simulink model "Main_ComplexTherma_Test_IGBT_Revised"  (R2022b)
settings: Solver=ode45  StartTime=0.0  StopTime=time  RelTol=1e-3  EnableMultiTasking=on
values from neighbouring files (symbols this model uses):
  C1diode = tau1diode/R1diode    (= 0.047619047619)    [fcnLE.m]
  C1igbt = tau1igbt/R1igbt    (= 0.0806451612903)    [fcnLE.m]
  C2diode = tau2diode/R2diode    (= 0.434782608696)    [fcnLE.m]
  C2igbt = tau2igbt/R2igbt    (= 0.909090909091)    [fcnLE.m]
  C3diode = tau3diode/R3diode    (= 1.27098321343)    [fcnLE.m]
  C3igbt = tau3igbt/R3igbt    (= 2.43697478992)    [fcnLE.m]
  C4diode = tau4diode/R4diode    (= 11.7824773414)    [fcnLE.m]
  C4igbt = tau4igbt/R4igbt    (= 11.8421052632)    [fcnLE.m]
  C5diode = tau5diode/R5diode    (= 237.037037037)    [fcnLE.m]
  C5igbt = tau5igbt/R5igbt    (= 219)    [fcnLE.m]
  fswitch = 10000    [fcnLE.m]
  R1diode = 0.0126    [fcnLE.m]
  R1igbt = 0.0062    [fcnLE.m]
  R2diode = 0.0391    [fcnLE.m]
  R2igbt = 0.022    [fcnLE.m]
  R3diode = 0.0417    [fcnLE.m]
  R3igbt = 0.0238    [fcnLE.m]
  R4diode = 0.0331    [fcnLE.m]
  R4igbt = 0.038    [fcnLE.m]
  R5diode = 0.0135    [fcnLE.m]
  R5igbt = 0.01    [fcnLE.m]
  R6igbt = 0.1    [fcnLE.m]
  udc = config_battery.U_sys_nom    [fcnLE.m]
undefined symbols (not defined in the file or in its folder): eqivalentCircuitParameters, eta_t, i_g, Rw, vehicle_weight
libraries: spsParallelRLCBranchLib x11, spsControlledCurrentSourceLib x2, spsVoltageMeasurementLib x2, spsDCVoltageSourceLib x1, spspowerguiLib x1
settings Model: Creator=fengqi.chang  LastModifiedBy=wangyifei
settings SolverCC: AlgebraicLoopSolver=TrustRegion
settings DataIOCC: LimitDataPoints=on  SaveFormat=Array  ReturnWorkspaceOutputs=off
settings OptimizationCC: LifeSpan=inf
settings DebuggingCC: SolverPrmCheckMsg=warning  UnconnectedInputMsg=warning  UnconnectedOutputMsg=warning  UnconnectedLineMsg=warning  SFUnexpectedBacktrackingDiag=warning  SFNoUnconditionalDefaultTransitionDiag=warning  SFExecutionAtInitializationDiag=none  SFMachineParentedDataDiag=warning  ArithmeticOperatorsInVariantConditions=warning
settings HardwareCC: ProdBitPerPointer=32  ProdBitPerSizeT=32  ProdBitPerPtrDiffT=32  ProdLargestAtomicFloat=None  ProdIntDivRoundTo=Undefined  ProdEndianess=Unspecified  ProdWordSize=32  ProdHWDeviceType=32-bit Generic
settings ModelReferenceCC: EnableRefExpFcnMdlSchedulingChecks=on  PropagateSignalLabelsOutOfModel=off
settings SFSimCC: SimUseLocalCustomCode=off  CustomCodeUndefinedFunction=UseInterfaceOnly
settings RTWCC: RTWUseLocalCustomCode=off
settings CodeAppCC: StateflowObjectComments=on
settings GRTTargetCC: TargetLangStandard=C89/C90 (ANSI)
settings ConfigComp: CovMetricSettings=dw  CovSaveCumulativeToWorkspaceVar=on  CovSaveSingleToWorkspaceVar=on  CovExternalEMLEnable=off  CovSFcnEnable=off
settings SimscapeCC: SimscapeNormalizeSystem=off

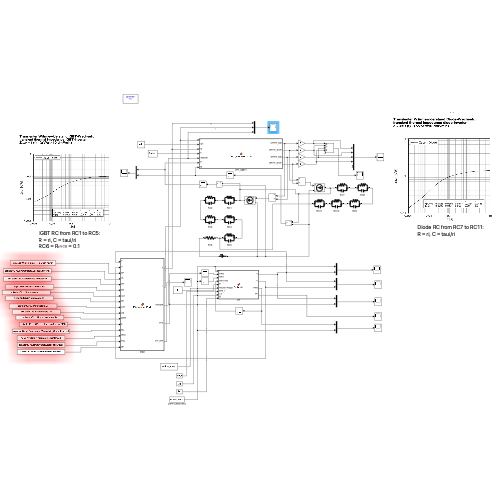
[thumbnail: Simulink's stored preview of the top-level diagram]
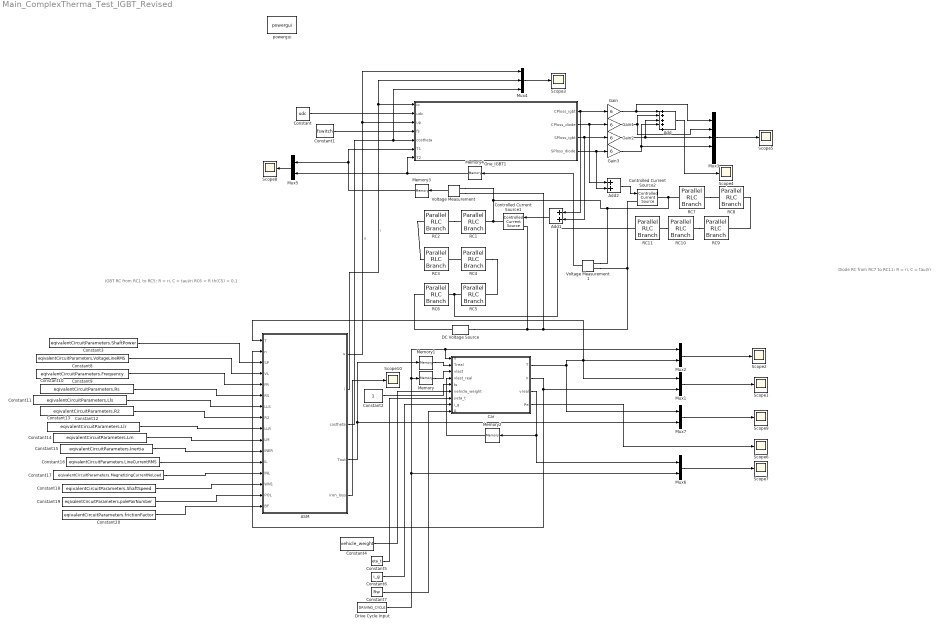
== system Main_ComplexTherma_Test_IGBT_Revised ==
  note: IGBT RC from RC1 to RC5:
      | R = ri, C = taui/ri
      | RC6 = R th(CS) = 0.1
  note: Diode RC from RC7 to RC11:
      | R = ri, C = taui/ri
  ASM : MATLAB Function  TreatAsAtomicUnit=on
  Add : Sum  Inputs=+++++
  Add1 : Sum
  Add2 : Sum
  Car : MATLAB Function  TreatAsAtomicUnit=on
  Constant : Constant  Value=udc
  Constant1 : Constant  Value=fswitch
  Constant10 : Constant  Value=eqivalentCircuitParameters.Rs
  Constant11 : Constant  Value=eqivalentCircuitParameters.Lls
  Constant12 : Constant  Value=eqivalentCircuitParameters.R2
  Constant13 : Constant  Value=eqivalentCircuitParameters.Llr
  Constant14 : Constant  Value=eqivalentCircuitParameters.Lm
  Constant15 : Constant  Value=eqivalentCircuitParameters.Inertia
  Constant16 : Constant  Value=eqivalentCircuitParameters.LineCurrentRMS
  Constant17 : Constant  Value=eqivalentCircuitParameters.MagnetizingCurrentNoLoad
  Constant18 : Constant  Value=eqivalentCircuitParameters.ShaftSpeed
  Constant19 : Constant  Value=eqivalentCircuitParameters.polePairNumber
  Constant2 : Constant
  Constant20 : Constant  Value=eqivalentCircuitParameters.frictionFactor
  Constant3 : Constant  Value=eqivalentCircuitParameters.ShaftPower
  Constant4 : Constant  Value=vehicle_weight
  Constant5 : Constant  Value=eta_t
  Constant6 : Constant  Value=i_g
  Constant7 : Constant  Value=Rw
  Constant8 : Constant  Value=eqivalentCircuitParameters.VoltageLineRMS
  Constant9 : Constant  Value=eqivalentCircuitParameters.Frequency
  Controlled Current Source1 : spsControlledCurrentSourceLib/Controlled Current Source  Initialize=on  Source_Type=AC  Amplitude=0  Phase=0  Frequency=0  Measurements=None
  Controlled Current Source2 : spsControlledCurrentSourceLib/Controlled Current Source  Initialize=on  Source_Type=AC  Amplitude=0  Phase=0  Frequency=0  Measurements=None
  DC Voltage Source : spsDCVoltageSourceLib/DC Voltage Source  Amplitude=50  Measurements=None
  Drive Cycle Input : FromWorkspace  VariableName=DRIVING_CYCLE  SampleTime=-1  OutputAfterFinalValue=Setting to zero
  Gain{,1..3} (4 alike) : Gain  Gain=6
  Memory : Memory  InheritSampleTime=on
  Memory1 : Memory  InheritSampleTime=on
  Memory2 : Memory  InheritSampleTime=on
  Memory3 : Memory  InitialCondition=25  InheritSampleTime=on
  Memory4 : Memory  InitialCondition=25  InheritSampleTime=on
  Mux{1..2,5..7} (5 alike) : Mux  Inputs=2
  Mux3 : Mux  Inputs=5
  Mux4 : Mux  Inputs=3
  One_IGBT1 : MATLAB Function  TreatAsAtomicUnit=on
  RC1 : spsParallelRLCBranchLib/Parallel RLC Branch  LConnTagsString=a  RConnTagsString=__new0  BranchType=RC  Resistance=R1igbt  Inductance=1e-3  SetiL0=off  InitialCurrent=0  Capacitance=C1igbt  Setx0=off  InitialVoltage=0  Measurements=None
  RC10 : spsParallelRLCBranchLib/Parallel RLC Branch  LConnTagsString=a  RConnTagsString=__new0  BranchType=RC  Resistance=R4diode  Inductance=1e-3  SetiL0=off  InitialCurrent=0  Capacitance=C4diode  Setx0=off  InitialVoltage=0  Measurements=None
  RC11 : spsParallelRLCBranchLib/Parallel RLC Branch  LConnTagsString=a  RConnTagsString=__new0  BranchType=RC  Resistance=R5diode  Inductance=1e-3  SetiL0=off  InitialCurrent=0  Capacitance=C5diode  Setx0=off  InitialVoltage=0  Measurements=None
  RC2 : spsParallelRLCBranchLib/Parallel RLC Branch  LConnTagsString=a  RConnTagsString=__new0  BranchType=RC  Resistance=R2igbt  Inductance=1e-3  SetiL0=off  InitialCurrent=0  Capacitance=C2igbt  Setx0=off  InitialVoltage=0  Measurements=None
  RC3 : spsParallelRLCBranchLib/Parallel RLC Branch  LConnTagsString=a  RConnTagsString=__new0  BranchType=RC  Resistance=R3igbt  Inductance=1e-3  SetiL0=off  InitialCurrent=0  Capacitance=C3igbt  Setx0=off  InitialVoltage=0  Measurements=None
  RC4 : spsParallelRLCBranchLib/Parallel RLC Branch  LConnTagsString=a  RConnTagsString=__new0  BranchType=RC  Resistance=R4igbt  Inductance=1e-3  SetiL0=off  InitialCurrent=0  Capacitance=C4igbt  Setx0=off  InitialVoltage=0  Measurements=None
  RC5 : spsParallelRLCBranchLib/Parallel RLC Branch  LConnTagsString=a  RConnTagsString=__new0  BranchType=RC  Resistance=R5igbt  Inductance=1e-3  SetiL0=off  InitialCurrent=0  Capacitance=C5igbt  Setx0=off  InitialVoltage=0  Measurements=None
  RC6 : spsParallelRLCBranchLib/Parallel RLC Branch  LConnTagsString=a  RConnTagsString=__new0  BranchType=R  Resistance=R6igbt  Inductance=1e-3  SetiL0=off  InitialCurrent=0  Capacitance=175  Setx0=on  InitialVoltage=0  Measurements=None
  RC7 : spsParallelRLCBranchLib/Parallel RLC Branch  LConnTagsString=a  RConnTagsString=__new0  BranchType=RC  Resistance=R1diode  Inductance=1e-3  SetiL0=off  InitialCurrent=0  Capacitance=C1diode  Setx0=off  InitialVoltage=0  Measurements=None
  RC8 : spsParallelRLCBranchLib/Parallel RLC Branch  LConnTagsString=a  RConnTagsString=__new0  BranchType=RC  Resistance=R2diode  Inductance=1e-3  SetiL0=off  InitialCurrent=0  Capacitance=C2diode  Setx0=off  InitialVoltage=0  Measurements=None
  RC9 : spsParallelRLCBranchLib/Parallel RLC Branch  LConnTagsString=a  RConnTagsString=__new0  BranchType=RC  Resistance=R3diode  Inductance=1e-3  SetiL0=off  InitialCurrent=0  Capacitance=C3diode  Setx0=off  InitialVoltage=0  Measurements=None
  Scope{1..10} (10 alike) : Scope
  Voltage Measurement : spsVoltageMeasurementLib/Voltage Measurement  PhasorSimulation=off  OutputType=Complex  PSBequivalent=0
  Voltage Measurement1 : spsVoltageMeasurementLib/Voltage Measurement  PhasorSimulation=off  OutputType=Complex  PSBequivalent=0
  powergui : spspowerguiLib/powergui  Priority=1  SimulationMode=Discrete  SampleTime=1  frequency=60  Iterations=50  frequencyindice=0  Pbase=100e6  ErrMax=1e-4  UnitsV=kV  UnitsW=MW  buscounter=0  FunctionMessages=off  echomessages=off  EnableUseOfTLC=off  CurrentSourceSwitches=off  DisableSnubberDevices=off  DisableRonSwitches=off  DisableVfSwitches=off  DisplayEquations=off  AutomaticDiscreteSolvers=off  SolverType=Backward Euler  Interpol=off  ExternalGateDelay=off  methode=off  Ts=100  x0status=blocks  SPID=off  SwTol=0  HookPort=off  NonlinearTolerance=1e-4  nMaxIteration=100  ContinueOnMaxIteration=off  RestoreLinks=warning  ResistiveCurrentMeasurement=off  Frange=[0:2:500]  Ylog=off  Xlog=on  ShowGrid=off  save=off  variable=ZData  structure=0  ZoomFFT=off  StartTime=0.0  cycles=1  DisplayStyle=1  fundamental=60  FreqAxis=off  MaxFrequency=1000  frequencyindicesteady=1  RmsSteady=1  display=off
  wires:
  Car/1(T) -> Mux1/1, ASM/1(T), Mux2/2, Mux7/1
  Car/2(n) -> ASM/2(n), Mux1/2
  Car/3(vreal) -> Mux6/1, Memory2/1
  ASM/3(costheta) -> One_IGBT1/5(costheta), Mux4/3
  Constant/1 -> One_IGBT1/2(udc)
  Constant1/1 -> One_IGBT1/4(fs)
  One_IGBT1/1(CPloss_igbt) -> Add1/1, Gain/1
  One_IGBT1/2(CPloss_diode) -> Add2/1, Gain1/1
  One_IGBT1/3(SPloss_igbt) -> Add1/2, Gain2/1
  One_IGBT1/4(SPloss_diode) -> Add2/2, Gain3/1
  Constant2/1 -> Car/5(ts)
  Gain/1 -> Mux3/1, Add/1
  Gain1/1 -> Mux3/2, Add/2
  Gain2/1 -> Mux3/3, Add/3
  Gain3/1 -> Add/4, Mux3/4
  Drive Cycle Input/1 -> Memory/1, Car/1(v), Mux2/1, Mux6/2
  ASM/4(Tout) -> Memory1/1, Mux7/2
  ASM/1(u) -> Mux4/1, One_IGBT1/3(up)  "u"
  Mux1/1 -> Scope1/1
  Memory1/1 -> Car/2(Treal)
  Mux2/1 -> Scope2/1
  Memory/1 -> Car/3(vlast)
  Memory2/1 -> Car/4(vlast_real)
  ASM/2(i) -> Mux4/2, One_IGBT1/1(io)  "i"
  Car/4(Pe) -> Scope6/1
  Add/1 -> Scope4/1
  Mux3/1 -> Scope5/1
  Mux4/1 -> Scope3/1
  Add1/1 -> Controlled Current Source1/1
  Voltage Measurement/1 -> Memory3/1
  Memory3/1 -> Mux5/1, One_IGBT1/6(T1)
  Add2/1 -> Controlled Current Source2/1
  Voltage Measurement1/1 -> Memory4/1
  Memory4/1 -> One_IGBT1/7(T2), Mux5/2
  Mux5/1 -> Scope8/1
  Mux6/1 -> Scope7/1
  Mux7/1 -> Scope9/1
  ASM/5(iron_loss) -> Scope10/1
  Constant4/1 -> Car/6(vehicle_weight)
  Constant5/1 -> Car/7(yeta_t)
  Constant6/1 -> Car/8(i_g)
  Constant7/1 -> Car/9(R)
  Constant3/1 -> ASM/3(SP)
  Constant8/1 -> ASM/4(VL)
  Constant9/1 -> ASM/5(FR)
  Constant10/1 -> ASM/6(RS)
  Constant11/1 -> ASM/7(LLS)
  Constant12/1 -> ASM/8(R2)
  Constant13/1 -> ASM/9(LLR)
  Constant14/1 -> ASM/10(LM)
  Constant15/1 -> ASM/11(INER)
  Constant16/1 -> ASM/12(IL)
  Constant17/1 -> ASM/13(INL)
  Constant18/1 -> ASM/14(WN1)
  Constant19/1 -> ASM/15(POL)
  Constant20/1 -> ASM/16(BF)
  connections:
  RC7/RConn1 -- Voltage Measurement/LConn1 -- RC1/RConn1 -- Controlled Current Source1/RConn1 -- Voltage Measurement1/LConn1 -- Controlled Current Source2/RConn1
  RC2/RConn1 -- RC1/LConn1
  RC2/LConn1 -- RC3/LConn1
  RC4/LConn1 -- RC3/RConn1
  RC4/RConn1 -- RC5/RConn1
  DC Voltage Source/RConn1 -- RC6/LConn1
  DC Voltage Source/LConn1 -- Controlled Current Source2/LConn1 -- Voltage Measurement1/LConn2 -- Voltage Measurement/LConn2 -- Controlled Current Source1/LConn1
  RC7/LConn1 -- RC8/RConn1
  RC8/LConn1 -- RC9/LConn1
  RC10/LConn1 -- RC9/RConn1
  RC11/LConn1 -- RC10/RConn1
  RC6/RConn1 -- RC11/RConn1 -- RC5/LConn1

== matlab function Main_ComplexTherma_Test_IGBT_Revised/ASM ==
  data: T input; n input; u output; i output; costheta output; Tout output; iron_loss output; SP input; VL input; FR input; RS input; LLS input; R2 input; LLR input; LM input; INER input; IL input; INL input; WN1 input; POL input; BF input
function [u,i,costheta,Tout,iron_loss] = ASMInverter_Pcalc(T,n, SP, VL, FR, RS, LLS, R2, LLR, LM, INER, IL, INL, WN1, POL, BF)
%%%%%%%%%%%%%%%%%%%%%%%Variable Table%%%%%%%%%%%%%%%%%%%%%%%%%%%%
%u          SQRT(3/2)*peak value of the output phase voltage from inverter    (V)
%i          SQRT(3/2)*peak value of the output phase current from inverter    (A)
%costheta   power factor required by the motor                      (none)
%T          torque required by the car                              (Nm)
%n          rotation speed of the motor required by the car         (rpm)
%%%%%%%%%%%%%%%%%%%%%%%%%%%%%%%%%%%%%%%%%%%%%%%%%%%%%%%%%%%%%%%%%
%%created in 2016 02 01 10 29
%%the model defines the interface of motor to inverter, which calculates 
%%the current, voltage as well as the power factor required by a motor.  
%%this model ignores the electrical transient status of the motor, but the error caused is unclear yet.
%%this model is only valid for induction motor. For more complex ones, model should be revised. 
%%%%%%%%%%%%%%%%%%%%  Parameters  %%%%%%%%%%%%%%%%%%%%%%
p = POL;
B = BF;
Lm = LM;
Lls = LLS;
Llr = LLR;
Ls = Lm + Lls;
Lr = Lm + Llr;
sigma = 1 - Lm^2/(Ls*Lr);
Rs = RS;
Rr = (Lm/(Lm + Llr))^2 * R2;
taur = Lr/Rr;
Prate = SP;
urate = VL;
fn = FR;
wm_n1 = WN1 * 2*pi/60;
wm_n2 = 12000 * 2*pi/60;     % ???
irate = IL;
i_noload = INL;
ir_dn = i_noload * sqrt(2); 
psis_dn = (sqrt(2)/sqrt(3)) * urate/(2*pi*fn);
psir_dn = psis_dn - (Ls*sigma) * ir_dn;
is_dn = psir_dn/Lm;
%%
%%%%%%%%%%%%%%%%%% input preparation %%%%%%%%%%%%%%%%%%%
%%%%%%%%%%%%%% no flux weakening required %%%%%%%%%%%%%%
wm = n/60 * 2*pi;
psir_d = psir_dn;
isd = is_dn;
Te = T + B*wm;
isq = Te/(3/2 * p * (Lm^2/Lr) * isd);
wr = p * wm;
wsl = Lm*isq/(taur*psir_d);
we = wr + wsl;
usd = Rs*isd - we*Ls*sigma*isq;
usq = Rs*isq + we*Ls*sigma*isd + we*(Lm/Lr)*psir_d;
i = sqrt(isq*isq+isd*isd);
u = sqrt(usq*usq+usd*usd);
costheta = (usd*isd+usq*isq)/u/i; % cos(atan(usq/usd)-atan(isq/isd));
Tout = T;
%%%%%%%%%%%%% if flux weakening required %%%%%%%%%%%%%%%
%%%%%%%%%%%%%%%%%%%%%%%   MA    %%%%%%%%%%%%%%%%%%%%%%%%
if wm > wm_n1 && wm <= wm_n2 || i > irate*sqrt(2) || u > urate*sqrt(2)
    if abs(n*T*2*pi/60) >= Prate
        Tout = Prate/(n/60*2*pi);
    else
        Tout = T;
    end
    psir_d_appr = psir_dn * wm_n1/wm;
    isd_appr = psir_d_appr/Lm;
    isq_appr = Te/(3/2 * p * (Lm^2/Lr) * isd_appr);
    wsl = Lm*isq_appr/(taur*psir_d_appr);
    we = wr + wsl;
    isd = isd_appr;
    isq = isq_appr;
%     isd = sqrt((((urate*sqrt(2))^2 / (we^2*Ls^2)) - (sigma^2 * (irate*sqrt(2))^2)) / (1-sigma^2));
%     psir_d = Lm*isd;
%     isq = Te/(3/2 * p * (Lm^2/Lr) * isd);
    usd = Rs*isd - we*Ls*sigma*isq;
    usq = Rs*isq + we*Ls*sigma*isd + we*(Lm/Lr)*psir_d;
%%%%%%%%%%%%%%%%%%%%%%   MTPF    %%%%%%%%%%%%%%%%%%%%%%%
elseif wm > wm_n2 || i > irate*sqrt(2) || u > urate*sqrt(2)
    if abs(n*T*2*pi/60) >= Prate
        Tout = Prate/(n/60*2*pi);
    else
        Tout = T;
    end
    psir_d_appr = psir_dn * wm_n2/wm;
    isd_appr = psir_d_appr/Lm;
    isq_appr = Te/(3/2 * p * (Lm^2/Lr) * isd_appr);
    wsl = Lm*isq_appr/(taur*psir_d_appr);
    we = wr + wsl;
    isd = isd_appr;
    isq = isq_appr;
%     isd = (urate*sqrt(2))/(sqrt(2)*we*Ls);
%     psir_d = Lm*isd;
%     isq = (urate*sqrt(2))/(sqrt(2)*we*Ls*sigma);
    usd = Rs*isd - we*Ls*sigma*isq;
    usq = Rs*isq + we*Ls*sigma*isd + we*(Lm/Lr)*psir_d;
end
i = sqrt(isq*isq+isd*isd);
u = sqrt(usq*usq+usd*usd);
costheta = (usd*isd+usq*isq)/u/i; % cos(atan(usq/usd)-atan(isq/isd));
%% iron loss caculation
% iron_loss = (9.128008725474993e-06*n^2 + 0.119030169537619*n)/3.3007*(abs(T)^0.5186);
beta = [7.47991049806284e-06,-0.00164430283336243,0.152741302836017,0.945215242366288];
iron_loss = (beta(1).*n.^2 + beta(2).*n).*beta(3).*(abs(T).^beta(4));
%%
if isnan(costheta)
    costheta = 1;
end
if n < 0.1 && T==0
    u = 0;
    i = 0;
    Tout = 0;
    costheta = 1;
end
if Tout ~= T
    Tout = T;
end

== matlab function Main_ComplexTherma_Test_IGBT_Revised/Car ==
  data: v input; T output; Treal input; vlast input; vlast_real input; ts input; n output; vreal output; Pe output; vehicle_weight input; yeta_t input; i_g input; R input
function [T,n,vreal,Pe] = CarModel(v,Treal,vlast,vlast_real,ts,vehicle_weight, yeta_t, i_g, R)
%%%%%%%%%%%%%%%%%%%%%%%%%%%%varialbe table%%%%%%%%%%%%%%%%%%%%%%%%%%%%%%%%%
%variavle name      meaning,                                             unit
%a,                 acceleration order of the car,                       (m/s^2)
%v,                 speed order of the car,                              (m/s)
%T,                 torque of the motor required by the car,             (Nm)
%n,                 rotation speed of the motor,                         (rpm)
%Pe,                power of the motor required by the car,              (kW)
%a_real,            real acceleration of the car,                        (m/s^2)
%vlast,             real speed of the car in last simulation period,     (m/s)
%nlast,             real rotation speed of the motor in last period,     (rad/s)
%Treal,             real torque from motor in  last simulation period,   (Nm)
%vnext,             real speed of the car,                               (m/s)
%ts,                simulation period,                                   (s)
%%%%%%%%%%%%%%%%%%%%%%%%%%%%%%%%%%%%%%%%%%%%%%%%%%%%%%%%%%%%%%%%%%%%%%%%%%%
%%%%%%%%%%%%%%%%%%%%%%%%%%%%parameter table%%%%%%%%%%%%%%%%%%%%%%%%%%%%%%%%
m=vehicle_weight;%1443.331;%1195;%                                  mass of the car,                      (kg)



a=(v-vlast)/ts;%calculate the acceleration needed in the next simulation period
if (vlast==0)&&(a==0)
    T=0;
else
    T = 1/yeta_t*(105.0138054720000+6.602356610980250*(vlast+v)/2+0.260513017636277*(vlast^2+v^2)/2+m*a)/(1/R*i_g);
    %parameters obtained from Agonne National Lab Testing Report
end
if (vlast==0)&&(Treal==0)
    areal=0;
else
    areal=(Treal*1/R*i_g*yeta_t-105.0138054720000-6.602356610980250*(vlast+v)/2-0.260513017636277*(vlast^2+v^2)/2)/(m);%calculate the real acceleration using Treal provided by the last simulation period
end
if(T<=0)&&(vlast_real<=0)
    T=0;
    areal=0;
end
vreal=vlast_real+areal*ts;%calculate the real speed in the next simulation period
n=(v+vlast)/2/R*i_g*30/pi;%calculate the real rotation speed in the next simulation period, in rpm
Pe=n*T/60*2*pi;%calculate the power needed in the next simulation period
end

== matlab function Main_ComplexTherma_Test_IGBT_Revised/One_IGBT1 ==
  data: io input; udc input; up input; fs input; CPloss_igbt output; CPloss_diode output; costheta input; SPloss_igbt output; SPloss_diode output; T1 input; T2 input
%%created in 2016 01 31 15 42
%%the model defines the input and output of the loss model of one switch
%%that is only the simplest version of an IGBT model
function [CPloss_igbt,CPloss_diode,SPloss_igbt,SPloss_diode] = IGBT_FS800R07A2E3(io,udc,up,fs,costheta,T1,T2)
%%this model is only for voltage source inverter or converter
%%%%%%%%%%%%%%%%%%%%%%%%%%%%parameter table%%%%%%%%%%%%%%%%%%%%%%%%%%%%%%%%
%%%%%%%%%%%%%%%%%%%%%%%%%%%%varialbe table%%%%%%%%%%%%%%%%%%%%%%%%%%%%%%%%%
%variavle name      meaning,                                                        unit
%io,                operation current, sqrt(3/2) peak value of phase current,       (A)
%up,                operation voltage, sqrt(3/2) peak value of phase voltage,       (V)
%udc,               DC bus voltage,                                                 (V)
%fs,                switching frequency,                                            (Hz)
%costheta,          power factor,                                                   (none)
%CPloss_igbt,       conduction loss on IGBT,                                        (W)
%CPloss_diode,      conduction loss on the reverse paralleled diode,                (W)
%SPloss_igbt,       switching loss on IGBT,                                         (W)
%SPloss_diode,      switching loss on the reverse paralleled diode,                 (W)
%%%%%%%%%%%%%%%%%%%%%%%%%%%%%%%%%%%%%%%%%%%%%%%%%%%%%%%%%%%%%%%%%%%%%%%%%%%
io=io/sqrt(3/2);
% uce=0.75-0.002*(T1-25);%@25degree, @150degress is 1.98V
% rc=0.85/600*(1+0.0052427*(T1-25));%
% udsat=0.8-0.002*(T2-25) ;%
% rd=0.6/400*(1+0.002*(T2-25));%

rc = 0.9/900*(1 + 0.0045*(T1 - 25))/4*3;  % 0.9/900*(1+0.0052427*(T1 - 25)); % resistor on the line and connection, usually ignored
rd = 0.6/400*(1 + 0.00167*(T2 - 25))/4*3; % 0.6/400*(1+0.002*(T2 - 25));     % resistor on the diode path, usually ignored
uce = 0.75 - 0.002*(T1 - 25);             % 0.75-0.002*(T1 - 25);            % @25degree, @150degress is 1.98V
udsat = 0.8 - 0.002*(T2 - 25);            % 0.8-0.002*(T2 - 25);%

m=up/sqrt(3/2)*2/udc; %modulation index

Eon_igbt=(0.011+0.0085/350*(abs(io)/4*3*(2/pi)-400))*((T1-125)*0.00129+1)/3*4;    % that is only the typical value, the value is influenced by T,r_gate and Ic
Eoff_igbt=(0.0175+0.0105/300*(abs(io)/4*3*(2/pi)-400))*((T1-125)*0.00148+1)/3*4;  % that is only the typical value, the value is influenced by T,r_gate and Ic
Eon_diode=0;          %that value is usually neglected
Eoff_diode=(0.007+0.0045/300*(abs(io)*(2/pi)/4*3-400))*((T2-125)*0.008571+1)/3*4; % that is only the typical value, the value is influenced by T,r_gate and Ic

CPloss_igbt=uce*abs(io)*(1/2/pi+m*costheta/8)+rc*io*io*(1/8+m*costheta/3/pi);
CPloss_diode=udsat*abs(io)*(1/2/pi-m*costheta/8)+rd*io*io*(1/8-m*costheta/3/pi);
SPloss_igbt=fs*(Eon_igbt+Eoff_igbt)/300*udc;
SPloss_diode=fs*(Eon_diode+Eoff_diode);
if(io==0)
    SPloss_igbt=0;
    SPloss_diode=0;
end
end
